simulink model "cluster_control"  (R2021b)
settings: Solver=ode3  StartTime=0.0  StopTime=inf  FixedStep=0.05  RelTol=1e-3
values from neighbouring files (symbols this model uses):
  grid_size = 1.0    (= 1)    [create_MatrixPlan.m]    (also in create_matrix.m)
  MatrixPlan = Grid.stat    [create_MatrixPlan.m]
  ThetaPlan = Grid.theta    [create_MatrixPlan.m]
  X = []    [create_MatrixPlan.m]    (also in create_matrix.m)
undefined symbols (not defined in the file or in its folder): DiscIntNeverNeededParam, Theta, Y
libraries: robotlib x3, spsEdgeDetectorLib x2, eeGeneralControl x2, robotcorelib x1, vrlib x1
settings Model: Creator=placido  LastModifiedBy=placido
settings OptimizationCC: DefaultParameterBehavior=Inlined  EnhancedBackFolding=on  PassReuseOutputArgsAs=Individual arguments  ZeroExternalMemoryAtStartup=off  ZeroInternalMemoryAtStartup=off  MaxStackSize=64  OptimizeBlockOrder=speed  DifferentSizesBufferReuse=on  OptimizationCustomize=off  EfficientTunableParamExpr=on
settings DebuggingCC: ParameterTunabilityLossMsg=error
settings HardwareCC: ProdBitPerPointer=32  ProdBitPerSizeT=32  ProdBitPerPtrDiffT=32  ProdLargestAtomicFloat=None  ProdIntDivRoundTo=Undefined  ProdEndianess=Unspecified  ProdWordSize=32  ProdHWDeviceType=Generic->Unspecified (assume 32-bit Generic)  UseEmbeddedCoderFeatures=off
settings SFSimCC: MATLABDynamicMemAlloc=off
settings RTWCC: Description=Embedded Coder  SystemTargetFile=ert.tlc  TemplateMakefile=ert_default_tmf  Toolchain=Catkin
settings CodeAppCC: ForceParamTrailComments=on  IgnoreCustomStorageClasses=off  OperatorAnnotations=on  SimulinkDataObjDesc=on  SFDataObjDesc=on  InsertBlockDesc=on
settings ERTTargetCC: SupportNonInlinedSFcns=on  ERTCustomFileTemplate=example_file_process.tlc

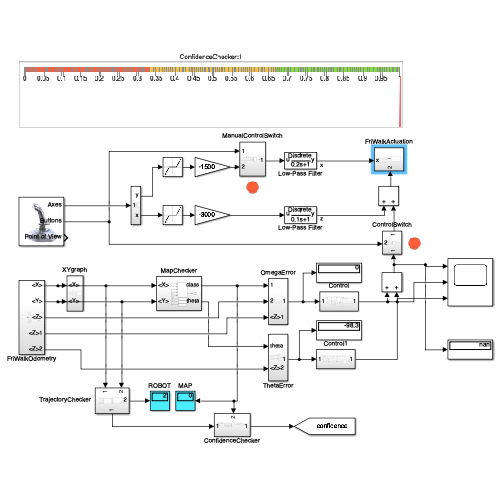
[thumbnail: Simulink's stored preview of the top-level diagram]
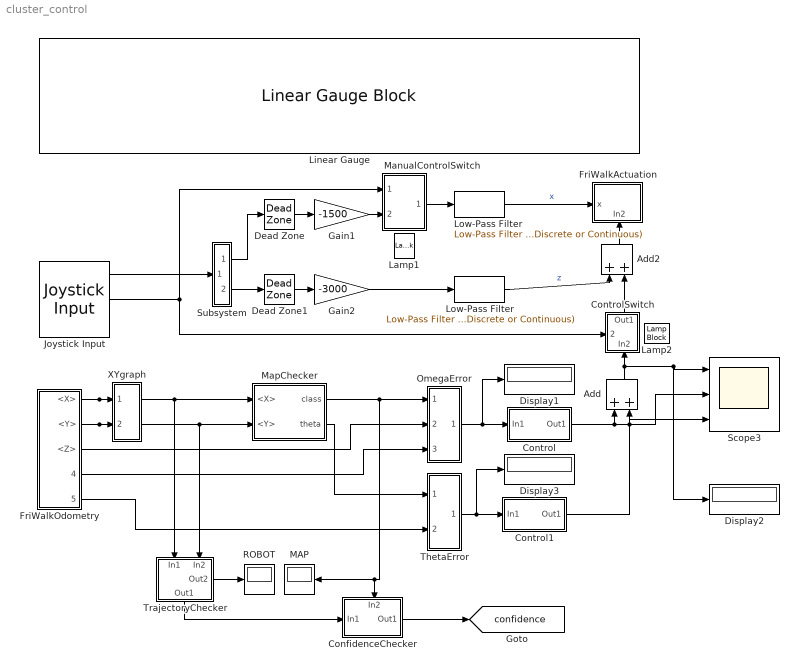
== system cluster_control ==
  Add : Sum
  Add2 : Sum
  ConfidenceChecker : Subsystem
      settings: PortSchema="{\"entries\":[{\"content\":{\"sides\":[{\"content\":{\"connectorIds\":[\"In1\"]},\"type\":\"ConnectorPlacement.EquallySpacedRectSide\",\"uuid\":\"736da283-826a-41a1-ab2f-9d6da9f5c537\"},{\"content\":{\"connectorIds\":[\"Out1\"],\"side\":\"RIGHT\"},\"type\":\"ConnectorPlacement.EquallySpacedRectSide\",\"uuid\":\"fb16d4a5-ef5f-46f9-a884-b772e060c9d5\"},{\"content\":{\"connectorIds\":[\"In2\"],\"side\":\"TOP\"},\"type\":\"ConnectorPlacement.EquallySpacedRectSide\",\"uuid\":\"bb3a1bcf-3e70-45c5-88c5-9ac1c74f7308\"}]},\"type\":\"ConnectorPlacement.EquallySpacedConnector\",\"uuid\":\"cba668bf-7104-4b4a-bb36-dc1117eda6ae\"}],\"packageUris\":[\"http://schema.mathworks.com/mf0/Connector/R2020b\"],\"version\":\"1.0\"}"
  Control : Subsystem
  Control1 : Subsystem
  ControlSwitch : Subsystem
      settings: PortSchema="{\"entries\":[{\"content\":{\"sides\":[{\"content\":{\"connectorIds\":[\"In1\"]},\"type\":\"ConnectorPlacement.EquallySpacedRectSide\",\"uuid\":\"736da283-826a-41a1-ab2f-9d6da9f5c537\"},{\"content\":{\"connectorIds\":[\"Out1\"],\"side\":\"RIGHT\"},\"type\":\"ConnectorPlacement.EquallySpacedRectSide\",\"uuid\":\"fb16d4a5-ef5f-46f9-a884-b772e060c9d5\"},{\"content\":{\"connectorIds\":[\"In2\"],\"side\":\"TOP\"},\"type\":\"ConnectorPlacement.EquallySpacedRectSide\",\"uuid\":\"bb3a1bcf-3e70-45c5-88c5-9ac1c74f7308\"}]},\"type\":\"ConnectorPlacement.EquallySpacedConnector\",\"uuid\":\"cba668bf-7104-4b4a-bb36-dc1117eda6ae\"}],\"packageUris\":[\"http://schema.mathworks.com/mf0/Connector/R2020b\"],\"version\":\"1.0\"}"
  Dead Zone : DeadZone  LowerValue=-0.05  UpperValue=0.05  SaturateOnIntegerOverflow=on
  Dead Zone1 : DeadZone  LowerValue=-0.05  UpperValue=0.05  SaturateOnIntegerOverflow=on
  Display1 : Display
  Display2 : Display
  Display3 : Display
  FriWalkActuation : Subsystem
      settings: PortSchema="{\"entries\":[{\"content\":{\"sides\":[{\"content\":{\"connectorIds\":[\"In1\"]},\"type\":\"ConnectorPlacement.EquallySpacedRectSide\",\"uuid\":\"fad886b0-8898-4bac-bc47-1487be3a8ce1\"},{\"content\":{\"connectorIds\":[],\"side\":\"RIGHT\"},\"type\":\"ConnectorPlacement.EquallySpacedRectSide\",\"uuid\":\"e9d1d614-549d-44a2-beba-90979377b2b4\"},{\"content\":{\"connectorIds\":[],\"side\":\"TOP\"},\"type\":\"ConnectorPlacement.EquallySpacedRectSide\",\"uuid\":\"ed6ed4f9-4387-46b5-862c-f90ba073a4c7\"},{\"content\":{\"connectorIds\":[\"In2\"],\"side\":\"BOTTOM\"},\"type\":\"ConnectorPlacement.EquallySpacedRectSide\",\"uuid\":\"7cfe686b-f408-46d9-a8bd-5284f8fc252e\"}]},\"type\":\"ConnectorPlacement.EquallySpacedConnector\",\"uuid\":\"116b1cd4-4c0e-47e3-bebf-f620f5773bae\"}],\"packageUris\":[\"http://schema.mathworks.com/mf0/Connector/R2020b\"],\"version\":\"1.0\"}"
  FriWalkOdometry : Subsystem
  Gain1 : Gain  Gain=-1500
  Gain2 : Gain  Gain=-3000
  Joystick Input : vrlib/Joystick Input  joyid=1  adjustports=on  forcefeed=off
  Lamp1 : LampBlock  LabelPosition=Hide
  Lamp2 : LampBlock  LabelPosition=Hide
  Linear Gauge : LinearGaugeBlock  ScaleMax=1
  Low-Pass Filter : eeGeneralControl/Low-Pass Filter (Discrete or Continuous)  K=1  T=0.1  B=inf  A=-inf  init_option=Inherited from block input  x0=0  Ts=-1
  "Low-Pass Filter " : eeGeneralControl/Low-Pass Filter (Discrete or Continuous)  K=1  T=0.2  B=inf  A=-inf  init_option=Inherited from block input  x0=0  Ts=-1
  MAP : Display
  ManualControlSwitch : Subsystem
  MapChecker : Subsystem
  OmegaError : Subsystem
  ROBOT : Display
  Scope3 : Scope  NumInputPorts=3
  Subsystem : Subsystem
  ThetaError : Subsystem
  TrajectoryChecker : Subsystem
      settings: PortSchema="{\"entries\":[{\"content\":{\"sides\":[{\"content\":{\"connectorIds\":[\"In1\",\"In2\"]},\"type\":\"ConnectorPlacement.EquallySpacedRectSide\",\"uuid\":\"f4d3361a-f3f4-4849-978b-67d63cd3eae6\"},{\"content\":{\"connectorIds\":[\"Out1\"],\"side\":\"RIGHT\"},\"type\":\"ConnectorPlacement.EquallySpacedRectSide\",\"uuid\":\"f98143c1-51f3-41c0-8490-df084dea68b1\"},{\"content\":{\"connectorIds\":[],\"side\":\"TOP\"},\"type\":\"ConnectorPlacement.EquallySpacedRectSide\",\"uuid\":\"080bcc7c-1926-46d7-b4f4-aa376e1645c9\"},{\"content\":{\"connectorIds\":[\"Out2\"],\"side\":\"BOTTOM\"},\"type\":\"ConnectorPlacement.EquallySpacedRectSide\",\"uuid\":\"0a09ebee-570f-48d0-979c-a1c6f9220c6d\"}]},\"type\":\"ConnectorPlacement.EquallySpacedConnector\",\"uuid\":\"b491dfc8-e398-4434-a831-abc9cadcaffe\"}],\"packageUris\":[\"http://schema.mathworks.com/mf0/Connector/R2020b\"],\"version\":\"1.0\"}"
  XYgraph : Subsystem
  tag scope: confidence=global
  wires:
  Dead Zone/1 -> Gain1/1
  Dead Zone1/1 -> Gain2/1
  Gain2/1 -> Low-Pass Filter/1
  Low-Pass Filter/1 -> Add2/1  "z"
  ControlSwitch/1(Out1) -> Add2/2
  Gain1/1 -> ManualControlSwitch/2(In2)
  Joystick Input/2 -> ControlSwitch/2(In3), ManualControlSwitch/1(In3)
  ManualControlSwitch/1(Out1) -> "Low-Pass Filter "/1
  Joystick Input/1 -> Subsystem/1(In1)
  Subsystem/1(y) -> Dead Zone/1
  Subsystem/2(x) -> Dead Zone1/1
  TrajectoryChecker/2(Out2) -> ROBOT/1
  MapChecker/1(class) -> ConfidenceChecker/2(In2), MAP/1, OmegaError/1(In1)
  TrajectoryChecker/1(Out1) -> ConfidenceChecker/1(In1)
  FriWalkOdometry/3(<Z>) -> OmegaError/2(In2)
  OmegaError/1(Out1) -> Control/1(In1), Display1/1
  "Low-Pass Filter "/1 -> FriWalkActuation/1(x)  "x"
  Add2/1 -> FriWalkActuation/2(In2)
  FriWalkOdometry/4(<Z>1) -> OmegaError/3(<Z>1)
  ConfidenceChecker/1(Out1) -> [confidence]
  FriWalkOdometry/2(<Y>) -> MapChecker/2(<Y>), TrajectoryChecker/2(In2), XYgraph/2(<Y>)
  FriWalkOdometry/1(<X>) -> XYgraph/1(<X>), MapChecker/1(<X>), TrajectoryChecker/1(In1)
  MapChecker/2(theta) -> ThetaError/1(theta)
  ThetaError/1(Out1) -> Display3/1, Control1/1(In1)
  Add/1 -> Display2/1, Scope3/1, ControlSwitch/1(In2)
  Control1/1(Out1) -> Scope3/3, Add/2
  FriWalkOdometry/5(<Z>2) -> ThetaError/2(<Z>2)
  Control/1(Out1) -> Scope3/2, Add/1

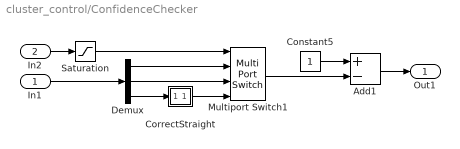
== system cluster_control/ConfidenceChecker ==
  In1 : Inport
  In2 : Inport  Port=2
  Add1 : Sum  Inputs=+-
  Constant5 : Constant
  CorrectStraight : Subsystem
  Demux : Demux  Outputs=3
  Multiport Switch1 : MultiPortSwitch
  Saturation : Saturate  UpperLimit=3  LowerLimit=1
  Out1 : Outport
  wires:
  Demux/1 -> Multiport Switch1/2
  Saturation/1 -> Multiport Switch1/1
  In2/1 -> Saturation/1
  In1/1 -> Demux/1
  Demux/2 -> Multiport Switch1/3
  Constant5/1 -> Add1/1
  Multiport Switch1/1 -> Add1/2
  Add1/1 -> Out1/1
  Demux/3 -> CorrectStraight/1(In1)
  CorrectStraight/1(Out1) -> Multiport Switch1/4

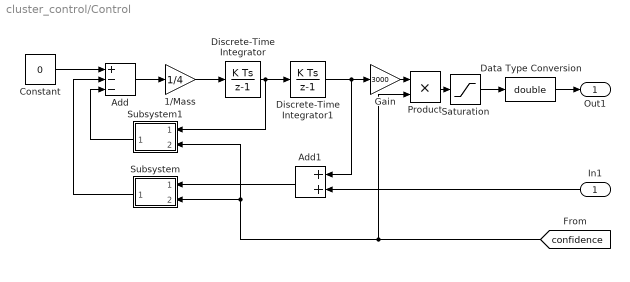
== system cluster_control/Control ==
  In1 : Inport
  1/Mass : Gain  Gain=1/4
  Add : Sum  Inputs=+--
  Add1 : Sum
  Constant : Constant  Value=0
  Data Type Conversion : DataTypeConversion  OutDataTypeStr=double
  Discrete-Time Integrator : DiscreteIntegrator  SampleTime=-1  ICPrevOutput=DiscIntNeverNeededParam  ICPrevScaledInput=DiscIntNeverNeededParam
  Discrete-Time Integrator1 : DiscreteIntegrator  SampleTime=-1  ICPrevOutput=DiscIntNeverNeededParam  ICPrevScaledInput=DiscIntNeverNeededParam
  Gain : Gain  Gain=3000
  Product : Product
  Saturation : Saturate  UpperLimit=4000  LowerLimit=-4000
  Subsystem : Subsystem
  Subsystem1 : Subsystem
  Out1 : Outport
  wires:
  Add/1 -> 1/Mass/1
  1/Mass/1 -> Discrete-Time Integrator/1
  Discrete-Time Integrator1/1 -> Gain/1, Add1/1
  Saturation/1 -> Data Type Conversion/1
  In1/1 -> Add1/2
  Constant/1 -> Add/1
  Gain/1 -> Product/1
  Add1/1 -> Subsystem/1(In1)
  [confidence] -> Product/2, Subsystem1/2(In2), Subsystem/2(In2)
  Subsystem/1(Out1) -> Add/2
  Subsystem1/1(Out1) -> Add/3
  Discrete-Time Integrator/1 -> Subsystem1/1(In1), Discrete-Time Integrator1/1
  Product/1 -> Saturation/1
  Data Type Conversion/1 -> Out1/1

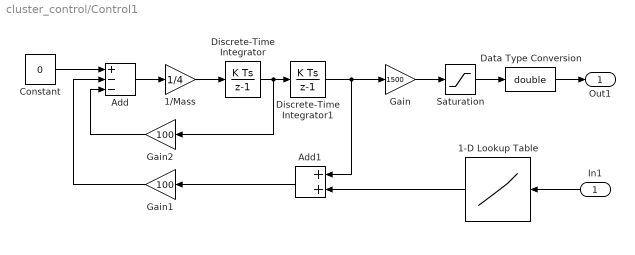
== system cluster_control/Control1 ==
  In1 : Inport
  1-D Lookup Table : Lookup_n-D  NumberOfTableDimensions=1  BreakpointsForDimension1=[-2:0.1:2]  Table=tanh([-4:0.2:4])  InternalRulePriority=Speed  RndMeth=Simplest  InputSameDT=on
  1/Mass : Gain  Gain=1/4
  Add : Sum  Inputs=+--
  Add1 : Sum
  Constant : Constant  Value=0
  Data Type Conversion : DataTypeConversion  OutDataTypeStr=double
  Discrete-Time Integrator : DiscreteIntegrator  SampleTime=-1  ICPrevOutput=DiscIntNeverNeededParam  ICPrevScaledInput=DiscIntNeverNeededParam
  Discrete-Time Integrator1 : DiscreteIntegrator  SampleTime=-1  ICPrevOutput=DiscIntNeverNeededParam  ICPrevScaledInput=DiscIntNeverNeededParam
  Gain : Gain  Gain=1500
  Gain1 : Gain  Gain=100
  Gain2 : Gain  Gain=100
  Saturation : Saturate  UpperLimit=2000  LowerLimit=-2000
  Out1 : Outport
  wires:
  Add/1 -> 1/Mass/1
  1/Mass/1 -> Discrete-Time Integrator/1
  Discrete-Time Integrator1/1 -> Gain/1, Add1/1
  Saturation/1 -> Data Type Conversion/1
  In1/1 -> 1-D Lookup Table/1
  Constant/1 -> Add/1
  Add1/1 -> Gain1/1
  Gain1/1 -> Add/2
  Gain2/1 -> Add/3
  Discrete-Time Integrator/1 -> Gain2/1, Discrete-Time Integrator1/1
  Gain/1 -> Saturation/1
  Data Type Conversion/1 -> Out1/1
  1-D Lookup Table/1 -> Add1/2

== system cluster_control/ControlSwitch ==
  In2 : Inport
  In3 : Inport  Port=2
  Constant : Constant  Value=0
  Multiport Switch1 : MultiPortSwitch  Inputs=2
  Subsystem : Subsystem
  Out1 : Outport
  wires:
  Multiport Switch1/1 -> Out1/1
  In2/1 -> Multiport Switch1/2
  In3/1 -> Subsystem/1(In1)
  Constant/1 -> Multiport Switch1/3
  Subsystem/1(Out1) -> Multiport Switch1/1

== system cluster_control/FriWalkActuation ==
  x : Inport
  In2 : Inport  Port=2
  FormatROSmsg : Subsystem
      settings: PortSchema="{\"entries\":[{\"content\":{\"sides\":[{\"content\":{\"connectorIds\":[\"In1\"]},\"type\":\"ConnectorPlacement.EquallySpacedRectSide\",\"uuid\":\"80db4c4e-b454-43dc-b812-026c7cc24cea\"},{\"content\":{\"connectorIds\":[\"Out1\"],\"side\":\"RIGHT\"},\"type\":\"ConnectorPlacement.EquallySpacedRectSide\",\"uuid\":\"0d8cdfbd-a1b4-4a02-a2d5-ca2aa92524dc\"},{\"content\":{\"connectorIds\":[],\"side\":\"TOP\"},\"type\":\"ConnectorPlacement.EquallySpacedRectSide\",\"uuid\":\"72419170-1751-49ac-a68b-d9f2c08aaa3e\"},{\"content\":{\"connectorIds\":[\"In2\"],\"side\":\"BOTTOM\"},\"type\":\"ConnectorPlacement.EquallySpacedRectSide\",\"uuid\":\"75ffd994-553f-4776-acb4-c5304dee729f\"}]},\"type\":\"ConnectorPlacement.EquallySpacedConnector\",\"uuid\":\"9d1dccf8-0b07-4894-830b-b51fe5199435\"}],\"packageUris\":[\"http://schema.mathworks.com/mf0/Connector/R2020b\"],\"version\":\"1.0\"}"
  Publish : robotlib/Publish  topicSource=Select from ROS network  topic=/cmd_current  messageType=geometry_msgs/Pose2D  legacyBusStruct=off  messageQueueLength=1
  wires:
  In2/1 -> FormatROSmsg/2(In2)
  x/1 -> FormatROSmsg/1(In1)
  FormatROSmsg/1(Out1) -> Publish/1

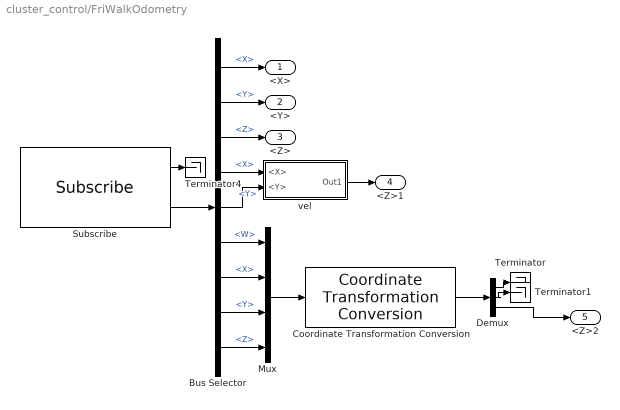
== system cluster_control/FriWalkOdometry ==
  Bus Selector : BusSelector  OutputSignals=Pose.Pose.Position.X,Pose.Pose.Position.Y,Twist.Twist.Angular.Z,Twist.Twist.Linear.X,Twist.Twist.Linear.Y,Pose.Pose.Orientation.W,Pose.Pose.Orientation.X,Pose.Pose.Orientation.Y,Pose.Pose.Orientation.Z
  Coordinate Transformation Conversion : robotcorelib/Coordinate Transformation Conversion  InputRepresentation=Quaternion  InputEulerSequence=ZYX  ShowTrVecInputPort=on  OutputRepresentation=Euler Angles  OutputEulerSequence=XYZ  ShowTrVecOutputPort=on  SimulateUsing=Interpreted execution
      settings: SourceProductBaseCode=NV,RO,RR,UV
  Demux : Demux  Outputs=3
  Mux : Mux
  Subscribe : robotlib/Subscribe  topicSource=Select from ROS network  topic=/odom  messageType=nav_msgs/Odometry  SampleTime=-1  legacyBusStruct=off  messageQueueLength=1
  Terminator : Terminator
  Terminator1 : Terminator
  Terminator4 : Terminator
  vel : Subsystem
  <X> : Outport
  <Y> : Outport  Port=2
  <Z> : Outport  Port=3
  <Z>1 : Outport  Port=4
  <Z>2 : Outport  Port=5
  wires:
  Bus Selector/3 -> <Z>/1  "<Z>"
  Subscribe/2 -> Bus Selector/1
  Bus Selector/2 -> <Y>/1  "<Y>"
  Bus Selector/1 -> <X>/1  "<X>"
  Subscribe/1 -> Terminator4/1
  Bus Selector/4 -> vel/1(<X>)  "<X>"
  Bus Selector/5 -> vel/2(<Y>)  "<Y>"
  vel/1(Out1) -> <Z>1/1
  Bus Selector/9 -> Mux/4  "<Z>"
  Bus Selector/8 -> Mux/3  "<Y>"
  Bus Selector/7 -> Mux/2  "<X>"
  Mux/1 -> Coordinate Transformation Conversion/1
  Coordinate Transformation Conversion/1 -> Demux/1
  Demux/1 -> Terminator/1
  Demux/2 -> Terminator1/1
  Demux/3 -> <Z>2/1
  Bus Selector/6 -> Mux/1  "<W>"

== system cluster_control/ManualControlSwitch ==
  In3 : Inport
  In2 : Inport  Port=2
  Constant : Constant  Value=0
  Multiport Switch1 : MultiPortSwitch  Inputs=2
  Subsystem : Subsystem
  Out1 : Outport
  wires:
  Multiport Switch1/1 -> Out1/1
  In2/1 -> Multiport Switch1/3
  In3/1 -> Subsystem/1(In1)
  Subsystem/1(Out1) -> Multiport Switch1/1
  Constant/1 -> Multiport Switch1/2

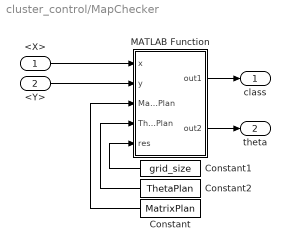
== system cluster_control/MapChecker ==
  <X> : Inport
  <Y> : Inport  Port=2
  Constant : Constant  Value=MatrixPlan
  Constant1 : Constant  Value=grid_size
  Constant2 : Constant  Value=ThetaPlan
  MATLAB Function : MATLAB Function  TreatAsAtomicUnit=on
  class : Outport
  theta : Outport  Port=2
  wires:
  MATLAB Function/1(out1) -> class/1
  <Y>/1 -> MATLAB Function/2(y)
  <X>/1 -> MATLAB Function/1(x)
  Constant1/1 -> MATLAB Function/5(res)
  Constant/1 -> MATLAB Function/3(MatrixPlan)
  MATLAB Function/2(out2) -> theta/1
  Constant2/1 -> MATLAB Function/4(ThetaPlan)

== system cluster_control/OmegaError ==
  In1 : Inport
  In2 : Inport  Port=2
  <Z>1 : Inport  Port=3
  Add : Sum  Inputs=-+
  OmegaGen : Subsystem
      settings: PortSchema="{\"entries\":[{\"content\":{\"sides\":[{\"content\":{\"connectorIds\":[\"In1\"]},\"type\":\"ConnectorPlacement.EquallySpacedRectSide\",\"uuid\":\"d127a8ec-93e7-471e-bbb0-066df5bdf07a\"},{\"content\":{\"connectorIds\":[\"Out1\"],\"side\":\"RIGHT\"},\"type\":\"ConnectorPlacement.EquallySpacedRectSide\",\"uuid\":\"ec8a3b2b-cd27-4e01-ad89-655080790167\"},{\"content\":{\"connectorIds\":[\"In2\"],\"side\":\"TOP\"},\"type\":\"ConnectorPlacement.EquallySpacedRectSide\",\"uuid\":\"59edb088-a787-43bf-9f00-32935fa10583\"}]},\"type\":\"ConnectorPlacement.EquallySpacedConnector\",\"uuid\":\"a91bf6c3-4289-4c51-ac92-f84d9e91c639\"}],\"packageUris\":[\"http://schema.mathworks.com/mf0/Connector/R2020b\"],\"version\":\"1.0\"}"
  Out1 : Outport
  wires:
  In1/1 -> OmegaGen/1(In1)
  Add/1 -> Out1/1
  In2/1 -> Add/2
  <Z>1/1 -> OmegaGen/2(<Z>1)
  OmegaGen/1(Out1) -> Add/1

== system cluster_control/Subsystem ==
  In1 : Inport
  Demux : Demux
  Terminator : Terminator
  Terminator3 : Terminator
  y : Outport
  x : Outport  Port=2
  wires:
  Demux/2 -> y/1  "x"
  Demux/3 -> x/1  "z"
  Demux/4 -> Terminator3/1
  In1/1 -> Demux/1
  Demux/1 -> Terminator/1

== system cluster_control/ThetaError ==
  theta : Inport
  <Z>2 : Inport  Port=2
  Add : Sum  Inputs=-+
  Out1 : Outport
  wires:
  Add/1 -> Out1/1
  <Z>2/1 -> Add/2
  theta/1 -> Add/1

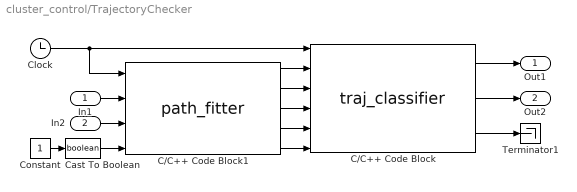
== system cluster_control/TrajectoryChecker ==
  In1 : Inport
  In2 : Inport  Port=2
  C/C++ Code Block : S-Function  FunctionName=traj_classifier  SFunctionModules=traj_classifier_wrapper  SFunctionDeploymentMode=off  EnableBusSupport=off  mask(S-Function Builder){}
      mask help: Simulink:masks:SFunctionBuilder_MD
      mask init:
      | val = [[.9  0.75 0.75 1 1 .9 .9 1]',[1 1 0.75 0.75 .9 .9 1 .9]'];try , sys = get_param(gcb,'SfunBuilderFcnName');if isempty(sys), sys = get_param(gcb,'FunctionName'); end,catch, sys = get_param(gcb,'FunctionName'); end
      settings: CopyFcn=set_param(gcbh,'LinkStatus','none')  OpenFcn=sfunctionwizard(gcbh)
      mask Display:
      | plot(val(:,1),val(:,2))
      | disp(sys)
      | port_label('input',1,'time')
      | port_label('input',2,'in_x')
      | port_label('input',3,'in_y')
      | port_label('input',4,'in_theta')
      | port_label('input',5,'in_kappa')
      | port_label('input',6,'in_valid')
      | port_label('output',1,'out_conf')
      | port_label('output',2,'out_class')
      | port_label('output',3,'out_valid')
  C/C++ Code Block1 : S-Function  FunctionName=path_fitter  SFunctionModules=path_fitter_wrapper smooth  SFunctionDeploymentMode=off  EnableBusSupport=off  mask(S-Function Builder){}
      mask help: Simulink:masks:SFunctionBuilder_MD
      mask init: same as cluster_control/TrajectoryChecker/C/C++ Code Block
      settings: CopyFcn=set_param(gcbh,'LinkStatus','none')  OpenFcn=sfunctionwizard(gcbh)
      mask Display:
      | plot(val(:,1),val(:,2))
      | disp(sys)
      | port_label('input',1,'time')
      | port_label('input',2,'in_x')
      | port_label('input',3,'in_y')
      | port_label('input',4,'in_valid')
      | port_label('output',1,'out_x')
      | port_label('output',2,'out_y')
      | port_label('output',3,'out_theta')
      | port_label('output',4,'out_kappa')
      | port_label('output',5,'out_valid')
  Cast To Boolean : DataTypeConversion  OutDataTypeStr=boolean
  Clock : Clock
  Constant : Constant
  Terminator1 : Terminator
  Out1 : Outport
  Out2 : Outport  Port=2
  wires:
  In1/1 -> C/C++ Code Block1/2
  C/C++ Code Block/2 -> Out2/1
  C/C++ Code Block/3 -> Terminator1/1
  C/C++ Code Block1/1 -> C/C++ Code Block/2
  Cast To Boolean/1 -> C/C++ Code Block1/4
  C/C++ Code Block1/4 -> C/C++ Code Block/5
  C/C++ Code Block1/3 -> C/C++ Code Block/4
  C/C++ Code Block1/2 -> C/C++ Code Block/3
  C/C++ Code Block1/5 -> C/C++ Code Block/6
  Clock/1 -> C/C++ Code Block1/1, C/C++ Code Block/1
  In2/1 -> C/C++ Code Block1/3
  C/C++ Code Block/1 -> Out1/1
  Constant/1 -> Cast To Boolean/1

== system cluster_control/XYgraph ==
  <X> : Inport
  <Y> : Inport  Port=2
  Add Constant : Bias  Bias=5
  Add Constant1 : Bias  Bias=5
  MATLAB Function : MATLAB Function  InitFcn=createFigureXY  TreatAsAtomicUnit=on
  wires:
  Add Constant/1 -> MATLAB Function/1(x)
  <X>/1 -> Add Constant/1
  Add Constant1/1 -> MATLAB Function/2(y)
  <Y>/1 -> Add Constant1/1

== system cluster_control/ConfidenceChecker/CorrectStraight ==
  In1 : Inport
  Gain : Gain  Gain=1.5
  Saturation1 : Saturate  UpperLimit=1  LowerLimit=0
  Out1 : Outport
  wires:
  In1/1 -> Gain/1
  Saturation1/1 -> Out1/1
  Gain/1 -> Saturation1/1

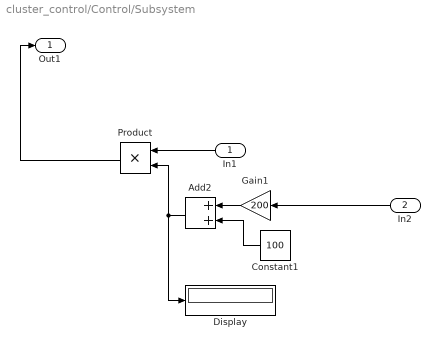
== system cluster_control/Control/Subsystem ==
  In1 : Inport
  In2 : Inport  Port=2
  Add2 : Sum
  Constant1 : Constant  Value=100
  Display : Display
  Gain1 : Gain  Gain=200
  Product : Product
  Out1 : Outport
  wires:
  In1/1 -> Product/1
  Product/1 -> Out1/1
  In2/1 -> Gain1/1
  Gain1/1 -> Add2/1
  Add2/1 -> Product/2, Display/1
  Constant1/1 -> Add2/2

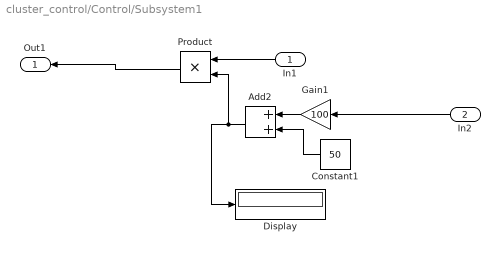
== system cluster_control/Control/Subsystem1 ==
  In1 : Inport
  In2 : Inport  Port=2
  Add2 : Sum
  Constant1 : Constant  Value=50
  Display : Display
  Gain1 : Gain  Gain=100
  Product : Product
  Out1 : Outport
  wires:
  In1/1 -> Product/1
  Product/1 -> Out1/1
  In2/1 -> Gain1/1
  Gain1/1 -> Add2/1
  Add2/1 -> Display/1, Product/2
  Constant1/1 -> Add2/2

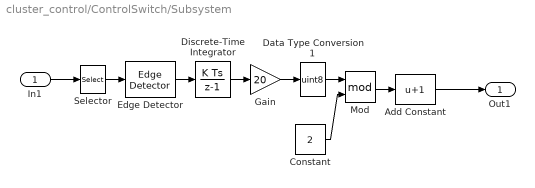
== system cluster_control/ControlSwitch/Subsystem ==
  In1 : Inport
  Add Constant : Bias  Bias=1
  Constant : Constant  Value=2  OutDataTypeStr=uint8
  Data Type Conversion1 : DataTypeConversion  OutDataTypeStr=uint8
  Discrete-Time Integrator : DiscreteIntegrator  SampleTime=-1  ICPrevOutput=DiscIntNeverNeededParam  ICPrevScaledInput=DiscIntNeverNeededParam
  Edge Detector : spsEdgeDetectorLib/Edge Detector  model=Rising  ic=0  Ts=0
      settings: SourceProductBaseCode=PS
  Gain : Gain  Gain=20
  Mod : Math  Operator=mod  SaturateOnIntegerOverflow=on
  Selector : Selector  InputPortWidth=17  IndexOptions=Index vector (dialog)  Indices=9  OutputSizes=1
  Out1 : Outport
  wires:
  In1/1 -> Selector/1
  Selector/1 -> Edge Detector/1
  Edge Detector/1 -> Discrete-Time Integrator/1
  Discrete-Time Integrator/1 -> Gain/1
  Gain/1 -> Data Type Conversion1/1
  Data Type Conversion1/1 -> Mod/1
  Constant/1 -> Mod/2
  Mod/1 -> Add Constant/1
  Add Constant/1 -> Out1/1

== system cluster_control/FriWalkActuation/FormatROSmsg ==
  In1 : Inport
  In2 : Inport  Port=2
  Blank Message : robotlib/Blank Message  messageClass=Message  entityType=geometry_msgs/Pose2D  messageType=geometry_msgs/Pose2D  SampleTime=inf  legacyBusStruct=off
  Bus Assignment : BusAssignment  AssignedSignals=Theta,X,Y
  Gain : Gain  Gain=0.6
  Out1 : Outport
  wires:
  Bus Assignment/1 -> Out1/1
  Blank Message/1 -> Bus Assignment/1
  In2/1 -> Bus Assignment/3, Gain/1
  In1/1 -> Bus Assignment/2
  Gain/1 -> Bus Assignment/4

== system cluster_control/FriWalkOdometry/vel ==
  <X> : Inport
  <Y> : Inport  Port=2
  Add : Sum
  Square : Math  Operator=square  SaturateOnIntegerOverflow=on
  Square Root : Sqrt  SaturateOnIntegerOverflow=on
  Square1 : Math  Operator=square  SaturateOnIntegerOverflow=on
  Out1 : Outport
  wires:
  <X>/1 -> Square/1
  Add/1 -> Square Root/1
  Square Root/1 -> Out1/1
  Square/1 -> Add/1
  <Y>/1 -> Square1/1
  Square1/1 -> Add/2

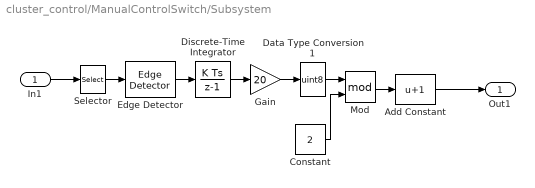
== system cluster_control/ManualControlSwitch/Subsystem ==
  In1 : Inport
  Add Constant : Bias  Bias=1
  Constant : Constant  Value=2  OutDataTypeStr=uint8
  Data Type Conversion1 : DataTypeConversion  OutDataTypeStr=uint8
  Discrete-Time Integrator : DiscreteIntegrator  SampleTime=-1  ICPrevOutput=DiscIntNeverNeededParam  ICPrevScaledInput=DiscIntNeverNeededParam
  Edge Detector : spsEdgeDetectorLib/Edge Detector  model=Rising  ic=0  Ts=0
      settings: SourceProductBaseCode=PS
  Gain : Gain  Gain=20
  Mod : Math  Operator=mod  SaturateOnIntegerOverflow=on
  Selector : Selector  InputPortWidth=17  IndexOptions=Index vector (dialog)  Indices=8  OutputSizes=1
  Out1 : Outport
  wires:
  In1/1 -> Selector/1
  Selector/1 -> Edge Detector/1
  Edge Detector/1 -> Discrete-Time Integrator/1
  Discrete-Time Integrator/1 -> Gain/1
  Gain/1 -> Data Type Conversion1/1
  Data Type Conversion1/1 -> Mod/1
  Constant/1 -> Mod/2
  Mod/1 -> Add Constant/1
  Add Constant/1 -> Out1/1

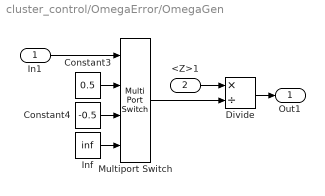
== system cluster_control/OmegaError/OmegaGen ==
  In1 : Inport
  <Z>1 : Inport  Port=2
  Constant3 : Constant  Value=0.5
  Constant4 : Constant  Value=-0.5
  Divide : Product  Inputs=*/
  Inf : Constant  Value=inf  OutDataTypeStr=Inherit: Inherit via back propagation
  Multiport Switch : MultiPortSwitch  DiagnosticForDefault=None
  Out1 : Outport
  wires:
  Inf/1 -> Multiport Switch/4
  Constant3/1 -> Multiport Switch/2
  In1/1 -> Multiport Switch/1
  Constant4/1 -> Multiport Switch/3
  Divide/1 -> Out1/1
  <Z>1/1 -> Divide/1
  Multiport Switch/1 -> Divide/2

== matlab function cluster_control/MapChecker/MATLAB Function ==
  data: x input; out1 output; y input; MatrixPlan input; ThetaPlan input; res input; out2 output
function [out1,out2] = checkState(x,y,MatrixPlan,ThetaPlan,res)

i=max(min(floor((x + 6)*res), size(MatrixPlan,1)),1);
j=max(min(floor((y + 6)*res), size(MatrixPlan,2)),1);

out1 = MatrixPlan(i, j);

out2 = ThetaPlan(i, j);

== matlab function cluster_control/XYgraph/MATLAB Function ==
  data: x input; y input
function fcn(x,y)

hold on
gca = plot(x,y,'.r');
